simulink model "DiscretePulseGenerator_TestGen4"  (R2017b)
settings: Solver=FixedStepDiscrete  StartTime=0.0  StopTime=10.0  RelTol=1e-3
undefined symbols (not defined in the file): Block_TestLib, trigger
settings Model: Creator=hbourbou  LastModifiedBy=hbourbou
settings DebuggingCC: ParameterOverflowMsg=none

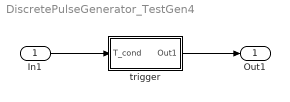
== system DiscretePulseGenerator_TestGen4 ==
  In1 : Inport
  trigger : Subsystem  AncestorBlock=Block_TestLib/trigger
  Out1 : Outport
  wires:
  In1/1 -> trigger/1(T_cond)
  trigger/1(Out1) -> Out1/1

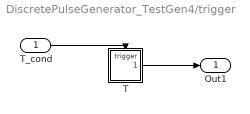
== system DiscretePulseGenerator_TestGen4/trigger ==
  T_cond : Inport  OutDataTypeStr=boolean
  T : Subsystem  TreatAsAtomicUnit=on
  Out1 : Outport
  wires:
  T_cond/1 -> T/Trigger
  T/1(Out1) -> Out1/1

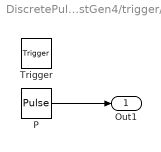
== system DiscretePulseGenerator_TestGen4/trigger/T ==
  Trigger : TriggerPort  VariantControl=Variant
  P : DiscretePulseGenerator  Amplitude=0.5  Period=5  PulseWidth=3  SampleTime=-1
  Out1 : Outport
  wires:
  P/1 -> Out1/1
